simulink model "calculator_using_switch"  (R2017b)
settings: Solver=FixedStepDiscrete  StartTime=0.0  StopTime=10.0  RelTol=1e-3
settings Model: Creator=ebrah  LastModifiedBy=ebrah
settings OptimizationCC: DefaultParameterBehavior=Inlined  PassReuseOutputArgsAs=Individual arguments
settings DebuggingCC: ParameterTunabilityLossMsg=error
settings SFSimCC: MATLABDynamicMemAlloc=off
settings RTWCC: SystemTargetFile=ert.tlc  GenCodeOnly=on  TemplateMakefile=ert_default_tmf  GenerateReport=on  IncludeHyperlinkInReport=on  LaunchReport=on  GenerateTraceInfo=on  GenerateTraceReport=on  GenerateTraceReportSl=on  GenerateTraceReportSf=on  GenerateTraceReportEml=on  GenerateWebview=on
settings CodeAppCC: ForceParamTrailComments=on  IgnoreCustomStorageClasses=off  OperatorAnnotations=on  SimulinkDataObjDesc=on  SFDataObjDesc=on  InsertBlockDesc=on
settings ERTTargetCC: TargetLangStandard=C99 (ISO)  GenerateSampleERTMain=on  InlinedParameterPlacement=NonHierarchical  ERTCustomFileTemplate=example_file_process.tlc

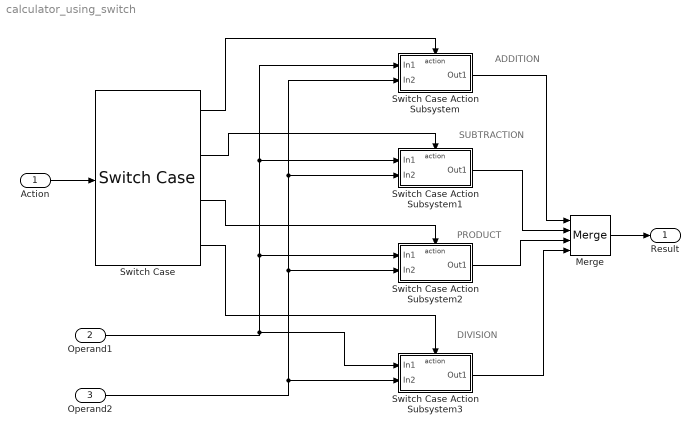
== system calculator_using_switch ==
  note: ADDITION
  note: SUBTRACTION
  note: PRODUCT
  note: DIVISION
  Action : Inport
  Operand1 : Inport  Port=2
  Operand2 : Inport  Port=3
  Merge : Merge  Inputs=4
  Switch Case : SwitchCase  CaseConditions={1,2,3,4}  ShowDefaultCase=off
  Switch Case Action Subsystem : Subsystem  TreatAsAtomicUnit=on
  Switch Case Action Subsystem1 : Subsystem  TreatAsAtomicUnit=on
  Switch Case Action Subsystem2 : Subsystem  TreatAsAtomicUnit=on
  Switch Case Action Subsystem3 : Subsystem  TreatAsAtomicUnit=on
  Result : Outport
  wires:
  Merge/1 -> Result/1
  Action/1 -> Switch Case/1
  Switch Case/1 -> Switch Case Action Subsystem/Action
  Switch Case/2 -> Switch Case Action Subsystem1/Action
  Switch Case/3 -> Switch Case Action Subsystem2/Action
  Switch Case/4 -> Switch Case Action Subsystem3/Action
  Operand1/1 -> Switch Case Action Subsystem3/1(In1), Switch Case Action Subsystem2/1(In1), Switch Case Action Subsystem1/1(In1), Switch Case Action Subsystem/1(In1)
  Operand2/1 -> Switch Case Action Subsystem3/2(In2), Switch Case Action Subsystem2/2(In2), Switch Case Action Subsystem1/2(In2), Switch Case Action Subsystem/2(In2)
  Switch Case Action Subsystem/1(Out1) -> Merge/1
  Switch Case Action Subsystem1/1(Out1) -> Merge/2
  Switch Case Action Subsystem2/1(Out1) -> Merge/3
  Switch Case Action Subsystem3/1(Out1) -> Merge/4

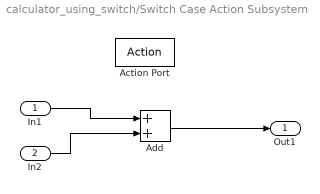
== system calculator_using_switch/Switch Case Action Subsystem ==
  In1 : Inport
  In2 : Inport  Port=2
  Action Port : ActionPort  ActionType=case
  Add : Sum
  Out1 : Outport
  wires:
  In1/1 -> Add/1
  In2/1 -> Add/2
  Add/1 -> Out1/1

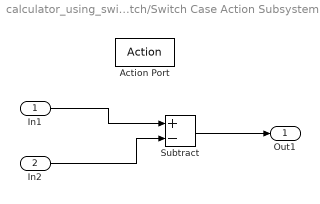
== system calculator_using_switch/Switch Case Action Subsystem1 ==
  In1 : Inport
  In2 : Inport  Port=2
  Action Port : ActionPort  ActionType=case
  Subtract : Sum  Inputs=+-
  Out1 : Outport
  wires:
  In1/1 -> Subtract/1
  In2/1 -> Subtract/2
  Subtract/1 -> Out1/1

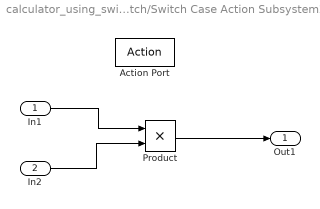
== system calculator_using_switch/Switch Case Action Subsystem2 ==
  In1 : Inport
  In2 : Inport  Port=2
  Action Port : ActionPort  ActionType=case
  Product : Product
  Out1 : Outport
  wires:
  In1/1 -> Product/1
  In2/1 -> Product/2
  Product/1 -> Out1/1

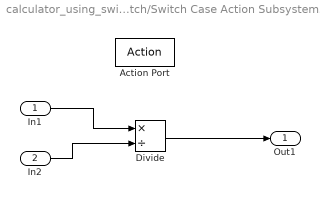
== system calculator_using_switch/Switch Case Action Subsystem3 ==
  In1 : Inport
  In2 : Inport  Port=2
  Action Port : ActionPort  ActionType=case
  Divide : Product  Inputs=*/
  Out1 : Outport
  wires:
  In1/1 -> Divide/1
  In2/1 -> Divide/2
  Divide/1 -> Out1/1
